simulink model "Full_Model_sim"  (R2022b)
settings: Solver=ode23t  StartTime=0.0  StopTime=1.5  RelTol=1e-3
values from neighbouring files (symbols this model uses):
  Ao = A - L*C    [Observer_Tune.m]
  Bo = [B L]    [Observer_Tune.m]
  Co = eye(3)    [Observer_Tune.m]
  Do = zeros(3, 3)    [Observer_Tune.m]
undefined symbols (not defined in the file or in its folder): bridge, diode, DiscIntNeverNeededParam, Discrete, Gamma, H, J, motor, Phi, pwr, Ri, Rw, sat, Time, uc
libraries: fl_lib x39, nesl_utility x27, ee_lib x25, simulink x3, ctrlSharedLib x1
(part 3 of 3)

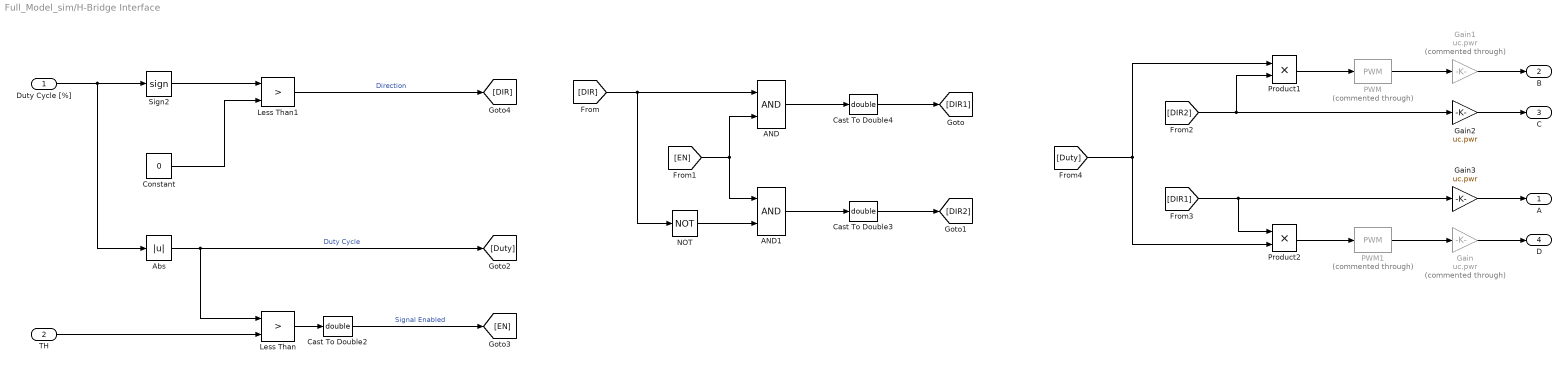
== system Full_Model_sim/H-Bridge Interface ==
  Duty Cycle [%] : Inport
  TH : Inport  Port=2
  AND : Logic  IconShape=distinctive  AllPortsSameDT=off  OutDataTypeStr=boolean
  AND1 : Logic  IconShape=distinctive  AllPortsSameDT=off  OutDataTypeStr=boolean
  Abs : Abs  SaturateOnIntegerOverflow=off
  Cast To Double2 : DataTypeConversion  OutDataTypeStr=double  SaturateOnIntegerOverflow=off  RndMeth=Floor
  Cast To Double3 : DataTypeConversion  OutDataTypeStr=double  SaturateOnIntegerOverflow=off  RndMeth=Floor
  Cast To Double4 : DataTypeConversion  OutDataTypeStr=double  SaturateOnIntegerOverflow=off  RndMeth=Floor
  Constant : Constant  Value=0
  Gain : Gain  Commented=through  Gain=uc.pwr
  Gain1 : Gain  Commented=through  Gain=uc.pwr
  Gain2 : Gain  Gain=uc.pwr
  Gain3 : Gain  Gain=uc.pwr
  Less Than : RelationalOperator  Operator=>  OutDataTypeStr=boolean  RndMeth=Simplest  InputSameDT=off
  Less Than1 : RelationalOperator  Operator=>  OutDataTypeStr=boolean  RndMeth=Simplest  InputSameDT=off
  NOT : Logic  Operator=NOT  IconShape=distinctive  AllPortsSameDT=off  OutDataTypeStr=boolean
  PWM : simulink/Discontinuities/PWM  Commented=through  DisableCoverage=on  Period=uc.Tpwm  InitialDelay=0  DisallowZeroDutyCycle=off  RunAtFixedTimeIntervals=on  SampleTime=uc.Tpwm/10
  PWM1 : simulink/Discontinuities/PWM  Commented=through  DisableCoverage=on  Period=uc.Tpwm  InitialDelay=0  DisallowZeroDutyCycle=off  RunAtFixedTimeIntervals=on  SampleTime=uc.Tpwm/10
  Product1 : Product
  Product2 : Product
  Sign2 : Signum
  A : Outport
  B : Outport  Port=2
  C : Outport  Port=3
  D : Outport  Port=4
  wires:
  TH/1 -> Less Than/2
  Duty Cycle [%]/1 -> Abs/1, Sign2/1
  Less Than/1 -> Cast To Double2/1
  Sign2/1 -> Less Than1/1
  Constant/1 -> Less Than1/2
  Abs/1 -> [Duty], Less Than/1  "Duty Cycle"
  Gain/1 -> D/1
  Gain1/1 -> B/1
  Gain2/1 -> C/1
  Gain3/1 -> A/1
  AND1/1 -> Cast To Double3/1
  AND/1 -> Cast To Double4/1
  NOT/1 -> AND1/2
  Product1/1 -> PWM/1
  Product2/1 -> PWM1/1
  Cast To Double2/1 -> [EN]  "Signal Enabled"
  Less Than1/1 -> [DIR]  "Direction"
  [DIR] -> NOT/1, AND/1
  [EN] -> AND/2, AND1/1
  Cast To Double4/1 -> [DIR1]
  Cast To Double3/1 -> [DIR2]
  [DIR2] -> Product1/2, Gain2/1
  [DIR1] -> Product2/1, Gain3/1
  [Duty] -> Product1/1, Product2/2
  PWM/1 -> Gain1/1
  PWM1/1 -> Gain/1

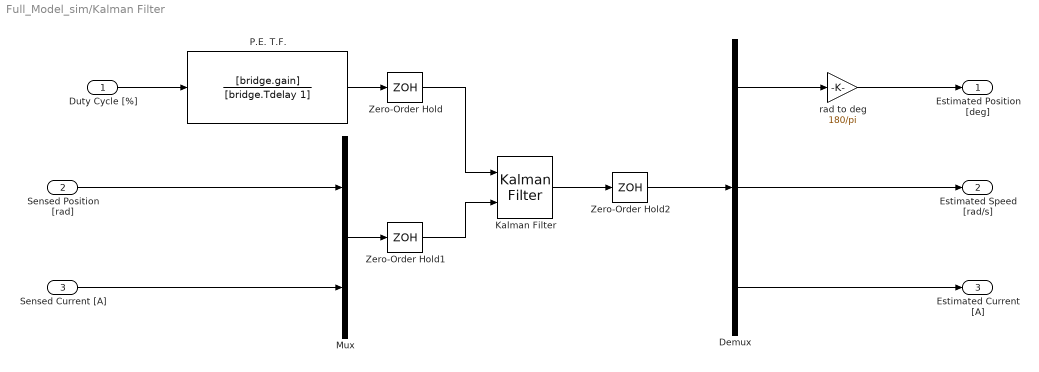
== system Full_Model_sim/Kalman Filter ==
  Duty Cycle [%] : Inport
  Sensed Position [rad] : Inport  Port=2
  Sensed Current [A] : Inport  Port=3
  Demux : Demux  Outputs=3
  Kalman Filter : ctrlSharedLib/Kalman Filter  TimeDomain=Discrete-Time  UseCurrentEstimator=on  ModelSource=Individual A, B, C, D matrices  ModelSourceVariable=ss(0.95,1,1,0,1)  A=Phi  B=Gamma  C=H  D=J  NumberOfStates=1  NumberOfInputs=1  NumberOfOutputs=1  InitialEstimateSource=Dialog  X0=0  P0=10  UseK=off  UseGH=off  NumberOfProcessNoiseInputs=1  G=1  TimeInvariantG=on  H=0  TimeInvariantH=on  Q=eye(3)  TimeInvariantQ=on  R=eye(2)  TimeInvariantR=on  N=0  TimeInvariantN=on  AddInputPort=on  AddEnablePort=off  OutputEstimatedY=off  OutputP=off  Ts=-1
  Mux : Mux  Inputs=2
  P.E. T.F. : TransferFcn  Numerator=[bridge.gain]  Denominator=[bridge.Tdelay 1]
  Zero-Order Hold : ZeroOrderHold  SampleTime=uc.Ts
  Zero-Order Hold1 : ZeroOrderHold  SampleTime=uc.Ts
  Zero-Order Hold2 : ZeroOrderHold  SampleTime=uc.Ts
  rad to deg : Gain  Gain=180/pi
  Estimated Position [deg] : Outport
  Estimated Speed [rad/s] : Outport  Port=2
  Estimated Current [A] : Outport  Port=3
  wires:
  Duty Cycle [%]/1 -> P.E. T.F./1
  Sensed Position [rad]/1 -> Mux/1
  Sensed Current [A]/1 -> Mux/2
  rad to deg/1 -> Estimated Position [deg]/1
  Demux/1 -> rad to deg/1
  Demux/3 -> Estimated Current [A]/1
  Demux/2 -> Estimated Speed [rad/s]/1
  Kalman Filter/1 -> Zero-Order Hold2/1
  Mux/1 -> Zero-Order Hold1/1
  P.E. T.F./1 -> Zero-Order Hold/1
  Zero-Order Hold/1 -> Kalman Filter/1
  Zero-Order Hold1/1 -> Kalman Filter/2
  Zero-Order Hold2/1 -> Demux/1

== system Full_Model_sim/Position Quantizer ==
  In : Inport
  Quantizer : Quantizer  QuantizationInterval=AS5600.q_rad
  Zero-Order Hold : ZeroOrderHold  Commented=through  SampleTime=uc.Ts
  Out : Outport
  wires:
  In/1 -> Quantizer/1
  Zero-Order Hold/1 -> Out/1
  Quantizer/1 -> Zero-Order Hold/1

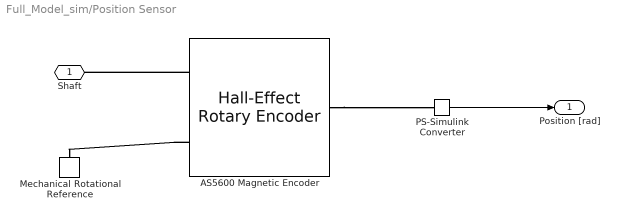
== system Full_Model_sim/Position Sensor ==
  AS5600 Magnetic Encoder : ee_lib/Sensors & Transducers/Hall-Effect Rotary Encoder  Ax=uc.pwr V  Ay=uc.pwr V  Vx0=0 V  Vy0=0 V  beta=0 deg  sensor_output=ee.enum.rotarysensors.output.decoded_ps  theta_specify=off  theta_priority=High  theta=180 deg  theta_nominal_specify=off  theta_nominal_unit=deg  theta_nominal_value=1
      settings: InternalSimscapePortConfiguration="{\"Bottom\":[],\"Left\":[{\"id\":\"R\",\"label\":\"R\",\"type\":\"foundation.mechanical.rotational.rotational\"},{\"id\":\"C\",\"label\":\"C\",\"type\":\"foundation.mechanical.rotational.rotational\"}],\"Right\":[{\"id\":\"A\",\"label\":\"Angle\",\"type\":\"output\"}],\"Top\":[]}"
  Mechanical Rotational Reference : fl_lib/Mechanical/Rotational Elements/Mechanical Rotational Reference
  PS-Simulink Converter : nesl_utility/PS-Simulink Converter  PhysicalDomain=network_engine_domain  SubClassName=ps_output  LeftPortType=input  RightPortType=output  PseudoPeriodic=off  Frequencies=[]  VectorFormat=inherit  Unit=inherit  AffineConversion=off
  Shaft : PMIOPort  Side=Left
  Position [rad] : Outport
  wires:
  PS-Simulink Converter/1 -> Position [rad]/1
  connections:
  AS5600 Magnetic Encoder/LConn2 -- Mechanical Rotational Reference/LConn1
  AS5600 Magnetic Encoder/RConn1 -- PS-Simulink Converter/LConn1
  AS5600 Magnetic Encoder/LConn1 -- Shaft/RConn1

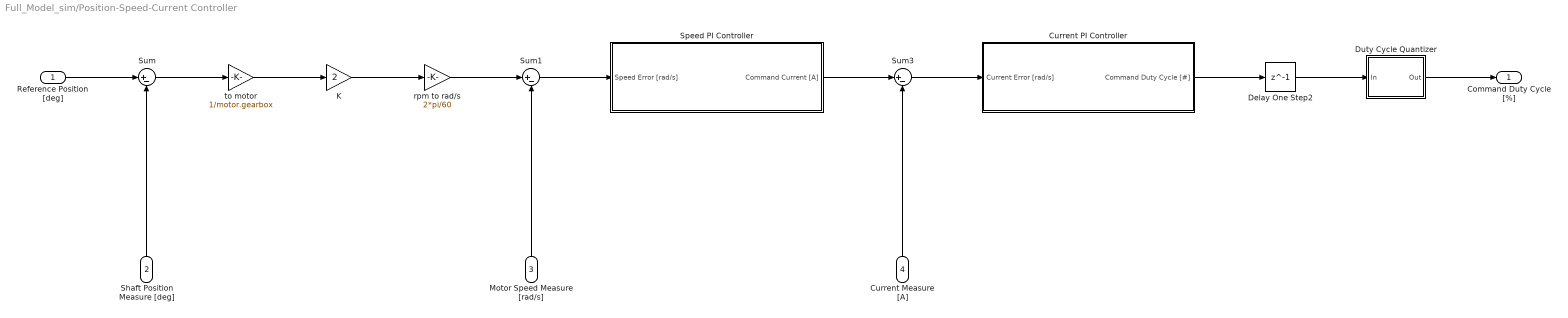
== system Full_Model_sim/Position-Speed-Current Controller ==
  Reference Position [deg] : Inport
  Shaft Position Measure [deg] : Inport  Port=2
  Motor Speed Measure [rad/s] : Inport  Port=3
  Current Measure [A] : Inport  Port=4
  Current PI Controller : Subsystem
  Delay One Step2 : Delay  DelayLength=1  SampleTime=uc.Ts
  Duty Cycle Quantizer : Subsystem
  K : Gain  Gain=2
  Speed PI Controller : Subsystem
  Sum : Sum  Inputs=|+-
  Sum1 : Sum  Inputs=|+-
  Sum3 : Sum  Inputs=|+-
  rpm to rad/s : Gain  Gain=2*pi/60
  to motor : Gain  Gain=1/motor.gearbox
  Command Duty Cycle [%] : Outport
  wires:
  Speed PI Controller/1(Command Current [A]) -> Sum3/1
  Current PI Controller/1(Command Duty Cycle [#]) -> Delay One Step2/1
  Sum3/1 -> Current PI Controller/1(Current Error [rad/s])
  Sum1/1 -> Speed PI Controller/1(Speed Error [rad/s])
  Shaft Position Measure [deg]/1 -> Sum/2
  Delay One Step2/1 -> Duty Cycle Quantizer/1(In)
  Duty Cycle Quantizer/1(Out) -> Command Duty Cycle [%]/1
  Current Measure [A]/1 -> Sum3/2
  Motor Speed Measure [rad/s]/1 -> Sum1/2
  to motor/1 -> K/1
  Reference Position [deg]/1 -> Sum/1
  K/1 -> rpm to rad/s/1
  Sum/1 -> to motor/1
  rpm to rad/s/1 -> Sum1/1

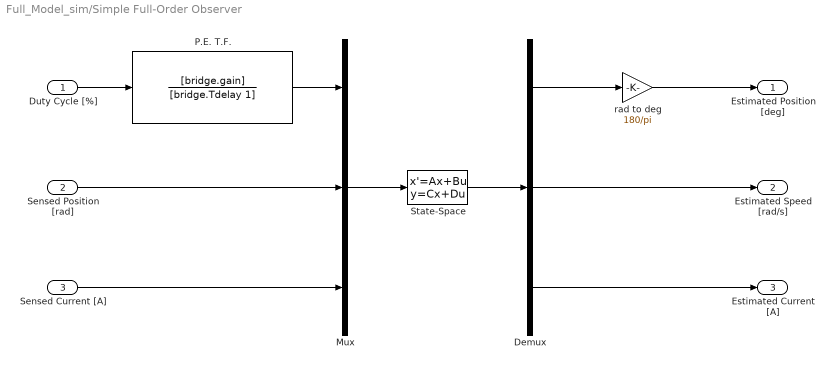
== system Full_Model_sim/Simple Full-Order Observer ==
  Duty Cycle [%] : Inport
  Sensed Position [rad] : Inport  Port=2
  Sensed Current [A] : Inport  Port=3
  Demux : Demux  Outputs=3
  Mux : Mux  Inputs=3
  P.E. T.F. : TransferFcn  Numerator=[bridge.gain]  Denominator=[bridge.Tdelay 1]
  State-Space : StateSpace  A=Ao  B=Bo  C=Co  D=Do  InitialCondition=0
  rad to deg : Gain  Gain=180/pi
  Estimated Position [deg] : Outport
  Estimated Speed [rad/s] : Outport  Port=2
  Estimated Current [A] : Outport  Port=3
  wires:
  Mux/1 -> State-Space/1
  P.E. T.F./1 -> Mux/1
  Demux/2 -> Estimated Speed [rad/s]/1
  Demux/3 -> Estimated Current [A]/1
  Demux/1 -> rad to deg/1
  rad to deg/1 -> Estimated Position [deg]/1
  Sensed Current [A]/1 -> Mux/3
  State-Space/1 -> Demux/1
  Sensed Position [rad]/1 -> Mux/2
  Duty Cycle [%]/1 -> P.E. T.F./1

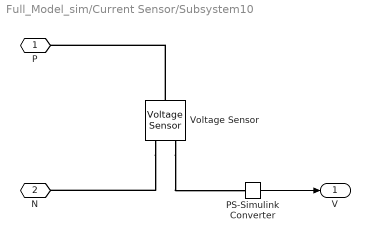
== system Full_Model_sim/Current Sensor/Subsystem10 ==
  PS-Simulink Converter : nesl_utility/PS-Simulink Converter  PhysicalDomain=network_engine_domain  SubClassName=ps_output  LeftPortType=input  RightPortType=output  PseudoPeriodic=off  Frequencies=[]  VectorFormat=inherit  Unit=inherit  AffineConversion=off
  Voltage Sensor : fl_lib/Electrical/Electrical Sensors/Voltage Sensor
  P : PMIOPort  Side=Left
  N : PMIOPort  Port=2  Side=Right
  V : Outport
  wires:
  PS-Simulink Converter/1 -> V/1
  connections:
  Voltage Sensor/RConn1 -- PS-Simulink Converter/LConn1
  Voltage Sensor/LConn1 -- P/RConn1
  Voltage Sensor/RConn2 -- N/RConn1

== system Full_Model_sim/H-Bridge/Subsystem1 ==
  PS-Simulink Converter : nesl_utility/PS-Simulink Converter  PhysicalDomain=network_engine_domain  SubClassName=ps_output  LeftPortType=input  RightPortType=output  PseudoPeriodic=off  Frequencies=[]  VectorFormat=inherit  Unit=inherit  AffineConversion=off
  Voltage Sensor : fl_lib/Electrical/Electrical Sensors/Voltage Sensor
  P : PMIOPort  Side=Left
  N : PMIOPort  Port=2  Side=Right
  V : Outport
  wires:
  PS-Simulink Converter/1 -> V/1
  connections:
  Voltage Sensor/RConn2 -- N/RConn1
  Voltage Sensor/LConn1 -- P/RConn1
  Voltage Sensor/RConn1 -- PS-Simulink Converter/LConn1

== system Full_Model_sim/H-Bridge/Subsystem10 ==
  PS-Simulink Converter : nesl_utility/PS-Simulink Converter  PhysicalDomain=network_engine_domain  SubClassName=ps_output  LeftPortType=input  RightPortType=output  PseudoPeriodic=off  Frequencies=[]  VectorFormat=inherit  Unit=inherit  AffineConversion=off
  Voltage Sensor : fl_lib/Electrical/Electrical Sensors/Voltage Sensor
  P : PMIOPort  Side=Left
  N : PMIOPort  Port=2  Side=Right
  V : Outport
  wires:
  PS-Simulink Converter/1 -> V/1
  connections:
  Voltage Sensor/RConn1 -- PS-Simulink Converter/LConn1
  Voltage Sensor/LConn1 -- P/RConn1
  Voltage Sensor/RConn2 -- N/RConn1

== system Full_Model_sim/H-Bridge/Subsystem11 ==
  Current Sensor : fl_lib/Electrical/Electrical Sensors/Current Sensor
  PS-Simulink Converter : nesl_utility/PS-Simulink Converter  PhysicalDomain=network_engine_domain  SubClassName=ps_output  LeftPortType=input  RightPortType=output  PseudoPeriodic=off  Frequencies=[]  VectorFormat=inherit  Unit=inherit  AffineConversion=off
  P : PMIOPort  Side=Left
  N : PMIOPort  Port=2  Side=Right
  I : Outport
  wires:
  PS-Simulink Converter/1 -> I/1
  connections:
  N/RConn1 -- Current Sensor/RConn2
  P/RConn1 -- Current Sensor/LConn1
  Current Sensor/RConn1 -- PS-Simulink Converter/LConn1

== system Full_Model_sim/H-Bridge/Subsystem12 ==
  PS-Simulink Converter : nesl_utility/PS-Simulink Converter  PhysicalDomain=network_engine_domain  SubClassName=ps_output  LeftPortType=input  RightPortType=output  PseudoPeriodic=off  Frequencies=[]  VectorFormat=inherit  Unit=inherit  AffineConversion=off
  Voltage Sensor : fl_lib/Electrical/Electrical Sensors/Voltage Sensor
  P : PMIOPort  Side=Left
  N : PMIOPort  Port=2  Side=Right
  V : Outport
  wires:
  PS-Simulink Converter/1 -> V/1
  connections:
  Voltage Sensor/RConn2 -- N/RConn1
  Voltage Sensor/LConn1 -- P/RConn1
  Voltage Sensor/RConn1 -- PS-Simulink Converter/LConn1

== system Full_Model_sim/H-Bridge/Subsystem13 ==
  Current Sensor : fl_lib/Electrical/Electrical Sensors/Current Sensor
  PS-Simulink Converter : nesl_utility/PS-Simulink Converter  PhysicalDomain=network_engine_domain  SubClassName=ps_output  LeftPortType=input  RightPortType=output  PseudoPeriodic=off  Frequencies=[]  VectorFormat=inherit  Unit=inherit  AffineConversion=off
  P : PMIOPort  Side=Left
  N : PMIOPort  Port=2  Side=Right
  I : Outport
  wires:
  PS-Simulink Converter/1 -> I/1
  connections:
  Current Sensor/RConn1 -- PS-Simulink Converter/LConn1
  P/RConn1 -- Current Sensor/LConn1
  N/RConn1 -- Current Sensor/RConn2

== system Full_Model_sim/H-Bridge/Subsystem14 ==
  Current Sensor : fl_lib/Electrical/Electrical Sensors/Current Sensor
  PS-Simulink Converter : nesl_utility/PS-Simulink Converter  PhysicalDomain=network_engine_domain  SubClassName=ps_output  LeftPortType=input  RightPortType=output  PseudoPeriodic=off  Frequencies=[]  VectorFormat=inherit  Unit=inherit  AffineConversion=off
  P : PMIOPort  Side=Left
  N : PMIOPort  Port=2  Side=Right
  I : Outport
  wires:
  PS-Simulink Converter/1 -> I/1
  connections:
  N/RConn1 -- Current Sensor/RConn2
  P/RConn1 -- Current Sensor/LConn1
  Current Sensor/RConn1 -- PS-Simulink Converter/LConn1

== system Full_Model_sim/H-Bridge/Subsystem15 ==
  Current Sensor : fl_lib/Electrical/Electrical Sensors/Current Sensor
  PS-Simulink Converter : nesl_utility/PS-Simulink Converter  PhysicalDomain=network_engine_domain  SubClassName=ps_output  LeftPortType=input  RightPortType=output  PseudoPeriodic=off  Frequencies=[]  VectorFormat=inherit  Unit=inherit  AffineConversion=off
  P : PMIOPort  Side=Left
  N : PMIOPort  Port=2  Side=Right
  I : Outport
  wires:
  PS-Simulink Converter/1 -> I/1
  connections:
  Current Sensor/RConn1 -- PS-Simulink Converter/LConn1
  P/RConn1 -- Current Sensor/LConn1
  N/RConn1 -- Current Sensor/RConn2

== system Full_Model_sim/H-Bridge/Subsystem16 ==
  PS-Simulink Converter : nesl_utility/PS-Simulink Converter  PhysicalDomain=network_engine_domain  SubClassName=ps_output  LeftPortType=input  RightPortType=output  PseudoPeriodic=off  Frequencies=[]  VectorFormat=inherit  Unit=inherit  AffineConversion=off
  Voltage Sensor : fl_lib/Electrical/Electrical Sensors/Voltage Sensor
  P : PMIOPort  Side=Left
  N : PMIOPort  Port=2  Side=Right
  V : Outport
  wires:
  PS-Simulink Converter/1 -> V/1
  connections:
  Voltage Sensor/RConn2 -- N/RConn1
  Voltage Sensor/LConn1 -- P/RConn1
  Voltage Sensor/RConn1 -- PS-Simulink Converter/LConn1

== system Full_Model_sim/H-Bridge/Subsystem2 ==
  PS-Simulink Converter : nesl_utility/PS-Simulink Converter  PhysicalDomain=network_engine_domain  SubClassName=ps_output  LeftPortType=input  RightPortType=output  PseudoPeriodic=off  Frequencies=[]  VectorFormat=inherit  Unit=inherit  AffineConversion=off
  Voltage Sensor : fl_lib/Electrical/Electrical Sensors/Voltage Sensor
  P : PMIOPort  Side=Left
  N : PMIOPort  Port=2  Side=Right
  V : Outport
  wires:
  PS-Simulink Converter/1 -> V/1
  connections:
  Voltage Sensor/RConn1 -- PS-Simulink Converter/LConn1
  Voltage Sensor/LConn1 -- P/RConn1
  Voltage Sensor/RConn2 -- N/RConn1

== system Full_Model_sim/H-Bridge/Subsystem3 ==
  Current Sensor : fl_lib/Electrical/Electrical Sensors/Current Sensor
  PS-Simulink Converter : nesl_utility/PS-Simulink Converter  PhysicalDomain=network_engine_domain  SubClassName=ps_output  LeftPortType=input  RightPortType=output  PseudoPeriodic=off  Frequencies=[]  VectorFormat=inherit  Unit=inherit  AffineConversion=off
  P : PMIOPort  Side=Left
  N : PMIOPort  Port=2  Side=Right
  I : Outport
  wires:
  PS-Simulink Converter/1 -> I/1
  connections:
  N/RConn1 -- Current Sensor/RConn2
  P/RConn1 -- Current Sensor/LConn1
  Current Sensor/RConn1 -- PS-Simulink Converter/LConn1

== system Full_Model_sim/H-Bridge/Subsystem4 ==
  PS-Simulink Converter : nesl_utility/PS-Simulink Converter  PhysicalDomain=network_engine_domain  SubClassName=ps_output  LeftPortType=input  RightPortType=output  PseudoPeriodic=off  Frequencies=[]  VectorFormat=inherit  Unit=inherit  AffineConversion=off
  Voltage Sensor : fl_lib/Electrical/Electrical Sensors/Voltage Sensor
  P : PMIOPort  Side=Left
  N : PMIOPort  Port=2  Side=Right
  V : Outport
  wires:
  PS-Simulink Converter/1 -> V/1
  connections:
  Voltage Sensor/RConn2 -- N/RConn1
  Voltage Sensor/LConn1 -- P/RConn1
  Voltage Sensor/RConn1 -- PS-Simulink Converter/LConn1

== system Full_Model_sim/H-Bridge/Subsystem5 ==
  PS-Simulink Converter : nesl_utility/PS-Simulink Converter  PhysicalDomain=network_engine_domain  SubClassName=ps_output  LeftPortType=input  RightPortType=output  PseudoPeriodic=off  Frequencies=[]  VectorFormat=inherit  Unit=inherit  AffineConversion=off
  Voltage Sensor : fl_lib/Electrical/Electrical Sensors/Voltage Sensor
  P : PMIOPort  Side=Left
  N : PMIOPort  Port=2  Side=Right
  V : Outport
  wires:
  PS-Simulink Converter/1 -> V/1
  connections:
  Voltage Sensor/RConn1 -- PS-Simulink Converter/LConn1
  Voltage Sensor/LConn1 -- P/RConn1
  Voltage Sensor/RConn2 -- N/RConn1

== system Full_Model_sim/H-Bridge/Subsystem6 ==
  PS-Simulink Converter : nesl_utility/PS-Simulink Converter  PhysicalDomain=network_engine_domain  SubClassName=ps_output  LeftPortType=input  RightPortType=output  PseudoPeriodic=off  Frequencies=[]  VectorFormat=inherit  Unit=inherit  AffineConversion=off
  Voltage Sensor : fl_lib/Electrical/Electrical Sensors/Voltage Sensor
  P : PMIOPort  Side=Left
  N : PMIOPort  Port=2  Side=Right
  V : Outport
  wires:
  PS-Simulink Converter/1 -> V/1
  connections:
  Voltage Sensor/RConn1 -- PS-Simulink Converter/LConn1
  Voltage Sensor/LConn1 -- P/RConn1
  Voltage Sensor/RConn2 -- N/RConn1

== system Full_Model_sim/H-Bridge/Subsystem7 ==
  Current Sensor : fl_lib/Electrical/Electrical Sensors/Current Sensor
  PS-Simulink Converter : nesl_utility/PS-Simulink Converter  PhysicalDomain=network_engine_domain  SubClassName=ps_output  LeftPortType=input  RightPortType=output  PseudoPeriodic=off  Frequencies=[]  VectorFormat=inherit  Unit=inherit  AffineConversion=off
  P : PMIOPort  Side=Left
  N : PMIOPort  Port=2  Side=Right
  I : Outport
  wires:
  PS-Simulink Converter/1 -> I/1
  connections:
  N/RConn1 -- Current Sensor/RConn2
  P/RConn1 -- Current Sensor/LConn1
  Current Sensor/RConn1 -- PS-Simulink Converter/LConn1

== system Full_Model_sim/H-Bridge/Subsystem8 ==
  Current Sensor : fl_lib/Electrical/Electrical Sensors/Current Sensor
  PS-Simulink Converter : nesl_utility/PS-Simulink Converter  PhysicalDomain=network_engine_domain  SubClassName=ps_output  LeftPortType=input  RightPortType=output  PseudoPeriodic=off  Frequencies=[]  VectorFormat=inherit  Unit=inherit  AffineConversion=off
  P : PMIOPort  Side=Left
  N : PMIOPort  Port=2  Side=Right
  I : Outport
  wires:
  PS-Simulink Converter/1 -> I/1
  connections:
  Current Sensor/RConn1 -- PS-Simulink Converter/LConn1
  P/RConn1 -- Current Sensor/LConn1
  N/RConn1 -- Current Sensor/RConn2

== system Full_Model_sim/H-Bridge/Subsystem9 ==
  Current Sensor : fl_lib/Electrical/Electrical Sensors/Current Sensor
  PS-Simulink Converter : nesl_utility/PS-Simulink Converter  PhysicalDomain=network_engine_domain  SubClassName=ps_output  LeftPortType=input  RightPortType=output  PseudoPeriodic=off  Frequencies=[]  VectorFormat=inherit  Unit=inherit  AffineConversion=off
  P : PMIOPort  Side=Left
  N : PMIOPort  Port=2  Side=Right
  I : Outport
  wires:
  PS-Simulink Converter/1 -> I/1
  connections:
  Current Sensor/RConn1 -- PS-Simulink Converter/LConn1
  P/RConn1 -- Current Sensor/LConn1
  N/RConn1 -- Current Sensor/RConn2

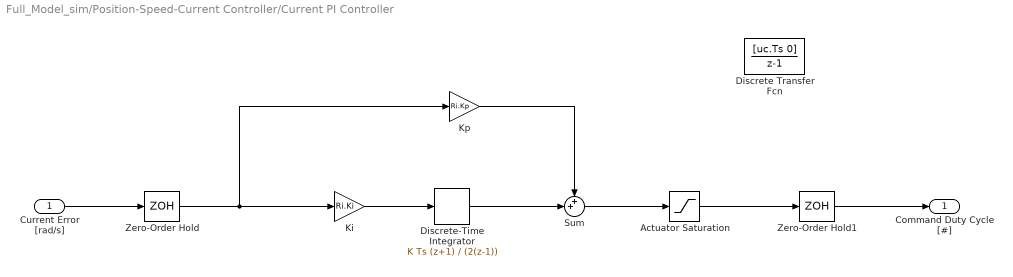
== system Full_Model_sim/Position-Speed-Current Controller/Current PI Controller ==
  Current Error [rad/s] : Inport
  Actuator Saturation : Saturate  UpperLimit=sat.d  LowerLimit=-sat.d
  Discrete Transfer Fcn : DiscreteTransferFcn  Numerator=[uc.Ts 0]  Denominator=[1 -1]  SampleTime=uc.Ts
  Discrete-Time Integrator : DiscreteIntegrator  IntegratorMethod=Integration: Trapezoidal  SampleTime=uc.Ts  ICPrevOutput=DiscIntNeverNeededParam  ICPrevScaledInput=DiscIntNeverNeededParam
  Ki : Gain  Gain=Ri.Ki
  Kp : Gain  Gain=Ri.Kp
  Sum : Sum  Inputs=++|
  Zero-Order Hold : ZeroOrderHold  SampleTime=uc.Ts
  Zero-Order Hold1 : ZeroOrderHold  SampleTime=uc.Ts
  Command Duty Cycle [#] : Outport
  wires:
  Discrete-Time Integrator/1 -> Sum/2
  Ki/1 -> Discrete-Time Integrator/1
  Sum/1 -> Actuator Saturation/1
  Kp/1 -> Sum/1
  Current Error [rad/s]/1 -> Zero-Order Hold/1
  Actuator Saturation/1 -> Zero-Order Hold1/1
  Zero-Order Hold/1 -> Kp/1, Ki/1
  Zero-Order Hold1/1 -> Command Duty Cycle [#]/1

== system Full_Model_sim/Position-Speed-Current Controller/Duty Cycle Quantizer ==
  In : Inport
  Quantizer : Quantizer  QuantizationInterval=uc.duty_step
  Zero-Order Hold : ZeroOrderHold  SampleTime=uc.Ts
  Out : Outport
  wires:
  Quantizer/1 -> Zero-Order Hold/1
  Zero-Order Hold/1 -> Out/1
  In/1 -> Quantizer/1

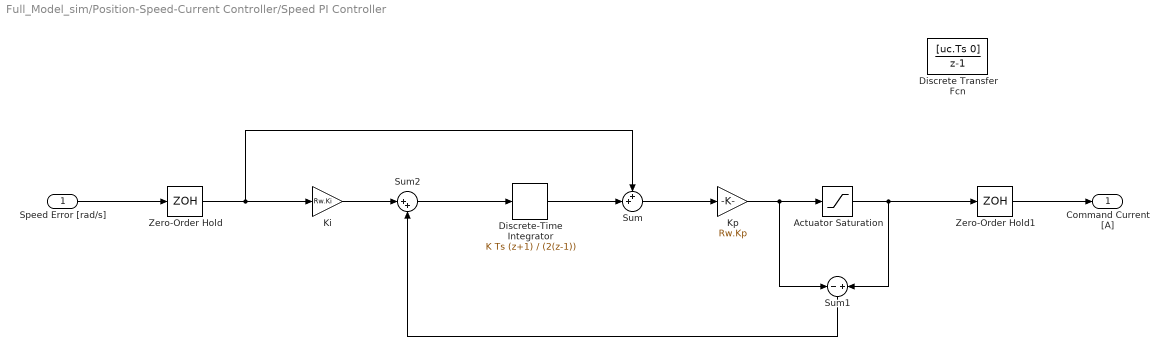
== system Full_Model_sim/Position-Speed-Current Controller/Speed PI Controller ==
  Speed Error [rad/s] : Inport
  Actuator Saturation : Saturate  UpperLimit=sat.I  LowerLimit=-sat.I
  Discrete Transfer Fcn : DiscreteTransferFcn  Numerator=[uc.Ts 0]  Denominator=[1 -1]  SampleTime=uc.Ts
  Discrete-Time Integrator : DiscreteIntegrator  IntegratorMethod=Integration: Trapezoidal  SampleTime=uc.Ts  ICPrevOutput=DiscIntNeverNeededParam  ICPrevScaledInput=DiscIntNeverNeededParam
  Ki : Gain  Gain=Rw.Ki
  Kp : Gain  Gain=Rw.Kp
  Sum : Sum  Inputs=++|
  Sum1 : Sum  Inputs=-+
  Sum2 : Sum  Inputs=|++
  Zero-Order Hold : ZeroOrderHold  SampleTime=uc.Ts
  Zero-Order Hold1 : ZeroOrderHold  SampleTime=uc.Ts
  Command Current [A] : Outport
  wires:
  Sum/1 -> Kp/1
  Sum1/1 -> Sum2/2
  Kp/1 -> Actuator Saturation/1, Sum1/1
  Speed Error [rad/s]/1 -> Zero-Order Hold/1
  Actuator Saturation/1 -> Zero-Order Hold1/1, Sum1/2
  Zero-Order Hold/1 -> Sum/1, Ki/1
  Zero-Order Hold1/1 -> Command Current [A]/1
  Sum2/1 -> Discrete-Time Integrator/1
  Discrete-Time Integrator/1 -> Sum/2
  Ki/1 -> Sum2/1
